simulink model "controllo_cartesiano"  (R2020b)
settings: Solver=VariableStepAuto  StartTime=0.0  StopTime=10.0  RelTol=1e-3
values from neighbouring files (symbols this model uses):
  f_G1 =     [workspaceMassaGravitaCoriolis.mat]
  f_G2 =     [workspaceMassaGravitaCoriolis.mat]
  f_G3 =     [workspaceMassaGravitaCoriolis.mat]
  f_M11 =     [workspaceMassaGravitaCoriolis.mat]
  f_M12 =     [workspaceMassaGravitaCoriolis.mat]
  f_M13 =     [workspaceMassaGravitaCoriolis.mat]
  f_M21 =     [workspaceMassaGravitaCoriolis.mat]
  f_M22 =     [workspaceMassaGravitaCoriolis.mat]
  f_M23 =     [workspaceMassaGravitaCoriolis.mat]
  f_M31 =     [workspaceMassaGravitaCoriolis.mat]
  f_M32 =     [workspaceMassaGravitaCoriolis.mat]
  f_M33 =     [workspaceMassaGravitaCoriolis.mat]
  f_V1 =     [workspaceMassaGravitaCoriolis.mat]
  f_V2 =     [workspaceMassaGravitaCoriolis.mat]
  f_V3 =     [workspaceMassaGravitaCoriolis.mat]
libraries: robotcorelib x1
(part 5 of 5)

== matlab function controllo_cartesiano/J ==
  data: Q input; dx output; dQ input; parametri input
function dx = J(Q,dQ,parametri)
l=parametri(1);
% d=parametri(2);
% m1=parametri(3);
% ma=parametri(4);
xc1=Q(1);
xc5=Q(2);
q2=Q(3);

J =[...
 
(l*sin(2*atan((2*l^2*sin(q2) + (3*l^4 + 4*cos(q2)*l^3*xc1 - 4*sin(q2)*l^3*xc5 - 2*cos(2*q2)*l^2*xc1^2 + 4*sin(2*q2)*l^2*xc1*xc5 + 2*cos(2*q2)*l^2*xc5^2 - 4*cos(q2)*l*xc1^3 + 4*sin(q2)*l*xc1^2*xc5 - 4*cos(q2)*l*xc1*xc5^2 + 4*sin(q2)*l*xc5^3 - xc1^4 - 2*xc1^2*xc5^2 - xc5^4)^(1/2) - 2*l*xc5)/(l^2 - 2*l*xc1 + xc1^2 + xc5^2 - 2*l^2*cos(q2) + 2*l*xc1*cos(q2) - 2*l*xc5*sin(q2))))*(((2*xc1 - 2*l + 2*l*cos(q2))*(2*l^2*sin(q2) + (3*l^4 + 4*cos(q2)*l^3*xc1 - 4*sin(q2)*l^3*xc5 - 2*cos(2*q2)*l^2*xc1^2 + 4*sin(2*q2)*l^2*xc1*xc5 + 2*cos(2*q2)*l^2*xc5^2 - 4*cos(q2)*l*xc1^3 + 4*sin(q2)*l*xc1^2*xc5 - 4*cos(q2)*l*xc1*xc5^2 + 4*sin(q2)*l*xc5^3 - xc1^4 - 2*xc1^2*xc5^2 - xc5^4)^(1/2) - 2*l*xc5))/(l^2 - 2*l*xc1 + xc1^2 + xc5^2 - 2*l^2*cos(q2) + 2*l*xc1*cos(q2) - 2*l*xc5*sin(q2))^2 + (2*(xc1 + l*cos(q2))*(- l^2 + 2*cos(q2)*l*xc1 - 2*sin(q2)*l*xc5 + xc1^2 + xc5^2))/((l^2 - 2*l*xc1 + xc1^2 + xc5^2 - 2*l^2*cos(q2) + 2*l*xc1*cos(q2) - 2*l*xc5*sin(q2))*(3*l^4 + 4*cos(q2)*l^3*xc1 - 4*sin(q2)*l^3*xc5 - 2*cos(2*q2)*l^2*xc1^2 + 4*sin(2*q2)*l^2*xc1*xc5 + 2*cos(2*q2)*l^2*xc5^2 - 4*cos(q2)*l*xc1^3 + 4*sin(q2)*l*xc1^2*xc5 - 4*cos(q2)*l*xc1*xc5^2 + 4*sin(q2)*l*xc5^3 - xc1^4 - 2*xc1^2*xc5^2 - xc5^4)^(1/2))))/((2*l^2*sin(q2) + (3*l^4 + 4*cos(q2)*l^3*xc1 - 4*sin(q2)*l^3*xc5 - 2*cos(2*q2)*l^2*xc1^2 + 4*sin(2*q2)*l^2*xc1*xc5 + 2*cos(2*q2)*l^2*xc5^2 - 4*cos(q2)*l*xc1^3 + 4*sin(q2)*l*xc1^2*xc5 - 4*cos(q2)*l*xc1*xc5^2 + 4*sin(q2)*l*xc5^3 - xc1^4 - 2*xc1^2*xc5^2 - xc5^4)^(1/2) - 2*l*xc5)^2/(l^2 - 2*l*xc1 + xc1^2 + xc5^2 - 2*l^2*cos(q2) + 2*l*xc1*cos(q2) - 2*l*xc5*sin(q2))^2 + 1) + 1, (l*sin(2*atan((2*l^2*sin(q2) + (3*l^4 + 4*cos(q2)*l^3*xc1 - 4*sin(q2)*l^3*xc5 - 2*cos(2*q2)*l^2*xc1^2 + 4*sin(2*q2)*l^2*xc1*xc5 + 2*cos(2*q2)*l^2*xc5^2 - 4*cos(q2)*l*xc1^3 + 4*sin(q2)*l*xc1^2*xc5 - 4*cos(q2)*l*xc1*xc5^2 + 4*sin(q2)*l*xc5^3 - xc1^4 - 2*xc1^2*xc5^2 - xc5^4)^(1/2) - 2*l*xc5)/(l^2 - 2*l*xc1 + xc1^2 + xc5^2 - 2*l^2*cos(q2) + 2*l*xc1*cos(q2) - 2*l*xc5*sin(q2))))*((2*l + (2*sin(q2)*l^3 - 2*sin(2*q2)*l^2*xc1 - 2*cos(2*q2)*l^2*xc5 - 2*sin(q2)*l*xc1^2 + 4*cos(q2)*l*xc1*xc5 - 6*sin(q2)*l*xc5^2 + 2*xc1^2*xc5 + 2*xc5^3)/(3*l^4 + 4*cos(q2)*l^3*xc1 - 4*sin(q2)*l^3*xc5 - 2*cos(2*q2)*l^2*xc1^2 + 4*sin(2*q2)*l^2*xc1*xc5 + 2*cos(2*q2)*l^2*xc5^2 - 4*cos(q2)*l*xc1^3 + 4*sin(q2)*l*xc1^2*xc5 - 4*cos(q2)*l*xc1*xc5^2 + 4*sin(q2)*l*xc5^3 - xc1^4 - 2*xc1^2*xc5^2 - xc5^4)^(1/2))/(l^2 - 2*l*xc1 + xc1^2 + xc5^2 - 2*l^2*cos(q2) + 2*l*xc1*cos(q2) - 2*l*xc5*sin(q2)) + ((2*xc5 - 2*l*sin(q2))*(2*l^2*sin(q2) + (3*l^4 + 4*cos(q2)*l^3*xc1 - 4*sin(q2)*l^3*xc5 - 2*cos(2*q2)*l^2*xc1^2 + 4*sin(2*q2)*l^2*xc1*xc5 + 2*cos(2*q2)*l^2*xc5^2 - 4*cos(q2)*l*xc1^3 + 4*sin(q2)*l*xc1^2*xc5 - 4*cos(q2)*l*xc1*xc5^2 + 4*sin(q2)*l*xc5^3 - xc1^4 - 2*xc1^2*xc5^2 - xc5^4)^(1/2) - 2*l*xc5))/(l^2 - 2*l*xc1 + xc1^2 + xc5^2 - 2*l^2*cos(q2) + 2*l*xc1*cos(q2) - 2*l*xc5*sin(q2))^2))/((2*l^2*sin(q2) + (3*l^4 + 4*cos(q2)*l^3*xc1 - 4*sin(q2)*l^3*xc5 - 2*cos(2*q2)*l^2*xc1^2 + 4*sin(2*q2)*l^2*xc1*xc5 + 2*cos(2*q2)*l^2*xc5^2 - 4*cos(q2)*l*xc1^3 + 4*sin(q2)*l*xc1^2*xc5 - 4*cos(q2)*l*xc1*xc5^2 + 4*sin(q2)*l*xc5^3 - xc1^4 - 2*xc1^2*xc5^2 - xc5^4)^(1/2) - 2*l*xc5)^2/(l^2 - 2*l*xc1 + xc1^2 + xc5^2 - 2*l^2*cos(q2) + 2*l*xc1*cos(q2) - 2*l*xc5*sin(q2))^2 + 1), - l*sin(q2) - (l*sin(2*atan((2*l^2*sin(q2) + (3*l^4 + 4*cos(q2)*l^3*xc1 - 4*sin(q2)*l^3*xc5 - 2*cos(2*q2)*l^2*xc1^2 + 4*sin(2*q2)*l^2*xc1*xc5 + 2*cos(2*q2)*l^2*xc5^2 - 4*cos(q2)*l*xc1^3 + 4*sin(q2)*l*xc1^2*xc5 - 4*cos(q2)*l*xc1*xc5^2 + 4*sin(q2)*l*xc5^3 - xc1^4 - 2*xc1^2*xc5^2 - xc5^4)^(1/2) - 2*l*xc5)/(l^2 - 2*l*xc1 + xc1^2 + xc5^2 - 2*l^2*cos(q2) + 2*l*xc1*cos(q2) - 2*l*xc5*sin(q2))))*((2*l^2*cos(q2) + (2*l*(- sin(q2)*l^2*xc1 - cos(q2)*l^2*xc5 + sin(2*q2)*l*xc1^2 + 2*cos(2*q2)*l*xc1*xc5 - sin(2*q2)*l*xc5^2 + sin(q2)*xc1^3 + cos(q2)*xc1^2*xc5 + sin(q2)*xc1*xc5^2 + cos(q2)*xc5^3))/(3*l^4 + 4*cos(q2)*l^3*xc1 - 4*sin(q2)*l^3*xc5 - 2*cos(2*q2)*l^2*xc1^2 + 4*sin(2*q2)*l^2*xc1*xc5 + 2*cos(2*q2)*l^2*xc5^2 - 4*cos(q2)*l*xc1^3 + 4*sin(q2)*l*xc1^2*xc5 - 4*cos(q2)*l*xc1*xc5^2 + 4*sin(q2)*l*xc5^3 - xc1^4 - 2*xc1^2*xc5^2 - xc5^4)^(1/2))/(l^2 - 2*l*xc1 + xc1^2 + xc5^2 - 2*l^2*cos(q2) + 2*l*xc1*cos(q2) - 2*l*xc5*sin(q2)) + (2*l*(xc5*cos(q2) - l*sin(q2) + xc1*sin(q2))*(2*l^2*sin(q2) + (3*l^4 + 4*cos(q2)*l^3*xc1 - 4*sin(q2)*l^3*xc5 - 2*cos(2*q2)*l^2*xc1^2 + 4*sin(2*q2)*l^2*xc1*xc5 + 2*cos(2*q2)*l^2*xc5^2 - 4*cos(q2)*l*xc1^3 + 4*sin(q2)*l*xc1^2*xc5 - 4*cos(q2)*l*xc1*xc5^2 + 4*sin(q2)*l*xc5^3 - xc1^4 - 2*xc1^2*xc5^2 - xc5^4)^(1/2) - 2*l*xc5))/(l^2 - 2*l*xc1 + xc1^2 + xc5^2 - 2*l^2*cos(q2) + 2*l*xc1*cos(q2) - 2*l*xc5*sin(q2))^2))/((2*l^2*sin(q2) + (3*l^4 + 4*cos(q2)*l^3*xc1 - 4*sin(q2)*l^3*xc5 - 2*cos(2*q2)*l^2*xc1^2 + 4*sin(2*q2)*l^2*xc1*xc5 + 2*cos(2*q2)*l^2*xc5^2 - 4*cos(q2)*l*xc1^3 + 4*sin(q2)*l*xc1^2*xc5 - 4*cos(q2)*l*xc1*xc5^2 + 4*sin(q2)*l*xc5^3 - xc1^4 - 2*xc1^2*xc5^2 - xc5^4)^(1/2) - 2*l*xc5)^2/(l^2 - 2*l*xc1 + xc1^2 + xc5^2 - 2*l^2*cos(q2) + 2*l*xc1*cos(q2) - 2*l*xc5*sin(q2))^2 + 1);...
    (l*cos(2*atan((2*l^2*sin(q2) + (3*l^4 + 4*cos(q2)*l^3*xc1 - 4*sin(q2)*l^3*xc5 - 2*cos(2*q2)*l^2*xc1^2 + 4*sin(2*q2)*l^2*xc1*xc5 + 2*cos(2*q2)*l^2*xc5^2 - 4*cos(q2)*l*xc1^3 + 4*sin(q2)*l*xc1^2*xc5 - 4*cos(q2)*l*xc1*xc5^2 + 4*sin(q2)*l*xc5^3 - xc1^4 - 2*xc1^2*xc5^2 - xc5^4)^(1/2) - 2*l*xc5)/(l^2 - 2*l*xc1 + xc1^2 + xc5^2 - 2*l^2*cos(q2) + 2*l*xc1*cos(q2) - 2*l*xc5*sin(q2))))*(((2*xc1 - 2*l + 2*l*cos(q2))*(2*l^2*sin(q2) + (3*l^4 + 4*cos(q2)*l^3*xc1 - 4*sin(q2)*l^3*xc5 - 2*cos(2*q2)*l^2*xc1^2 + 4*sin(2*q2)*l^2*xc1*xc5 + 2*cos(2*q2)*l^2*xc5^2 - 4*cos(q2)*l*xc1^3 + 4*sin(q2)*l*xc1^2*xc5 - 4*cos(q2)*l*xc1*xc5^2 + 4*sin(q2)*l*xc5^3 - xc1^4 - 2*xc1^2*xc5^2 - xc5^4)^(1/2) - 2*l*xc5))/(l^2 - 2*l*xc1 + xc1^2 + xc5^2 - 2*l^2*cos(q2) + 2*l*xc1*cos(q2) - 2*l*xc5*sin(q2))^2 + (2*(xc1 + l*cos(q2))*(- l^2 + 2*cos(q2)*l*xc1 - 2*sin(q2)*l*xc5 + xc1^2 + xc5^2))/((l^2 - 2*l*xc1 + xc1^2 + xc5^2 - 2*l^2*cos(q2) + 2*l*xc1*cos(q2) - 2*l*xc5*sin(q2))*(3*l^4 + 4*cos(q2)*l^3*xc1 - 4*sin(q2)*l^3*xc5 - 2*cos(2*q2)*l^2*xc1^2 + 4*sin(2*q2)*l^2*xc1*xc5 + 2*cos(2*q2)*l^2*xc5^2 - 4*cos(q2)*l*xc1^3 + 4*sin(q2)*l*xc1^2*xc5 - 4*cos(q2)*l*xc1*xc5^2 + 4*sin(q2)*l*xc5^3 - xc1^4 - 2*xc1^2*xc5^2 - xc5^4)^(1/2))))/((2*l^2*sin(q2) + (3*l^4 + 4*cos(q2)*l^3*xc1 - 4*sin(q2)*l^3*xc5 - 2*cos(2*q2)*l^2*xc1^2 + 4*sin(2*q2)*l^2*xc1*xc5 + 2*cos(2*q2)*l^2*xc5^2 - 4*cos(q2)*l*xc1^3 + 4*sin(q2)*l*xc1^2*xc5 - 4*cos(q2)*l*xc1*xc5^2 + 4*sin(q2)*l*xc5^3 - xc1^4 - 2*xc1^2*xc5^2 - xc5^4)^(1/2) - 2*l*xc5)^2/(l^2 - 2*l*xc1 + xc1^2 + xc5^2 - 2*l^2*cos(q2) + 2*l*xc1*cos(q2) - 2*l*xc5*sin(q2))^2 + 1), (l*cos(2*atan((2*l^2*sin(q2) + (3*l^4 + 4*cos(q2)*l^3*xc1 - 4*sin(q2)*l^3*xc5 - 2*cos(2*q2)*l^2*xc1^2 + 4*sin(2*q2)*l^2*xc1*xc5 + 2*cos(2*q2)*l^2*xc5^2 - 4*cos(q2)*l*xc1^3 + 4*sin(q2)*l*xc1^2*xc5 - 4*cos(q2)*l*xc1*xc5^2 + 4*sin(q2)*l*xc5^3 - xc1^4 - 2*xc1^2*xc5^2 - xc5^4)^(1/2) - 2*l*xc5)/(l^2 - 2*l*xc1 + xc1^2 + xc5^2 - 2*l^2*cos(q2) + 2*l*xc1*cos(q2) - 2*l*xc5*sin(q2))))*((2*l + (2*sin(q2)*l^3 - 2*sin(2*q2)*l^2*xc1 - 2*cos(2*q2)*l^2*xc5 - 2*sin(q2)*l*xc1^2 + 4*cos(q2)*l*xc1*xc5 - 6*sin(q2)*l*xc5^2 + 2*xc1^2*xc5 + 2*xc5^3)/(3*l^4 + 4*cos(q2)*l^3*xc1 - 4*sin(q2)*l^3*xc5 - 2*cos(2*q2)*l^2*xc1^2 + 4*sin(2*q2)*l^2*xc1*xc5 + 2*cos(2*q2)*l^2*xc5^2 - 4*cos(q2)*l*xc1^3 + 4*sin(q2)*l*xc1^2*xc5 - 4*cos(q2)*l*xc1*xc5^2 + 4*sin(q2)*l*xc5^3 - xc1^4 - 2*xc1^2*xc5^2 - xc5^4)^(1/2))/(l^2 - 2*l*xc1 + xc1^2 + xc5^2 - 2*l^2*cos(q2) + 2*l*xc1*cos(q2) - 2*l*xc5*sin(q2)) + ((2*xc5 - 2*l*sin(q2))*(2*l^2*sin(q2) + (3*l^4 + 4*cos(q2)*l^3*xc1 - 4*sin(q2)*l^3*xc5 - 2*cos(2*q2)*l^2*xc1^2 + 4*sin(2*q2)*l^2*xc1*xc5 + 2*cos(2*q2)*l^2*xc5^2 - 4*cos(q2)*l*xc1^3 + 4*sin(q2)*l*xc1^2*xc5 - 4*cos(q2)*l*xc1*xc5^2 + 4*sin(q2)*l*xc5^3 - xc1^4 - 2*xc1^2*xc5^2 - xc5^4)^(1/2) - 2*l*xc5))/(l^2 - 2*l*xc1 + xc1^2 + xc5^2 - 2*l^2*cos(q2) + 2*l*xc1*cos(q2) - 2*l*xc5*sin(q2))^2))/((2*l^2*sin(q2) + (3*l^4 + 4*cos(q2)*l^3*xc1 - 4*sin(q2)*l^3*xc5 - 2*cos(2*q2)*l^2*xc1^2 + 4*sin(2*q2)*l^2*xc1*xc5 + 2*cos(2*q2)*l^2*xc5^2 - 4*cos(q2)*l*xc1^3 + 4*sin(q2)*l*xc1^2*xc5 - 4*cos(q2)*l*xc1*xc5^2 + 4*sin(q2)*l*xc5^3 - xc1^4 - 2*xc1^2*xc5^2 - xc5^4)^(1/2) - 2*l*xc5)^2/(l^2 - 2*l*xc1 + xc1^2 + xc5^2 - 2*l^2*cos(q2) + 2*l*xc1*cos(q2) - 2*l*xc5*sin(q2))^2 + 1),   l*cos(q2) - (l*cos(2*atan((2*l^2*sin(q2) + (3*l^4 + 4*cos(q2)*l^3*xc1 - 4*sin(q2)*l^3*xc5 - 2*cos(2*q2)*l^2*xc1^2 + 4*sin(2*q2)*l^2*xc1*xc5 + 2*cos(2*q2)*l^2*xc5^2 - 4*cos(q2)*l*xc1^3 + 4*sin(q2)*l*xc1^2*xc5 - 4*cos(q2)*l*xc1*xc5^2 + 4*sin(q2)*l*xc5^3 - xc1^4 - 2*xc1^2*xc5^2 - xc5^4)^(1/2) - 2*l*xc5)/(l^2 - 2*l*xc1 + xc1^2 + xc5^2 - 2*l^2*cos(q2) + 2*l*xc1*cos(q2) - 2*l*xc5*sin(q2))))*((2*l^2*cos(q2) + (2*l*(- sin(q2)*l^2*xc1 - cos(q2)*l^2*xc5 + sin(2*q2)*l*xc1^2 + 2*cos(2*q2)*l*xc1*xc5 - sin(2*q2)*l*xc5^2 + sin(q2)*xc1^3 + cos(q2)*xc1^2*xc5 + sin(q2)*xc1*xc5^2 + cos(q2)*xc5^3))/(3*l^4 + 4*cos(q2)*l^3*xc1 - 4*sin(q2)*l^3*xc5 - 2*cos(2*q2)*l^2*xc1^2 + 4*sin(2*q2)*l^2*xc1*xc5 + 2*cos(2*q2)*l^2*xc5^2 - 4*cos(q2)*l*xc1^3 + 4*sin(q2)*l*xc1^2*xc5 - 4*cos(q2)*l*xc1*xc5^2 + 4*sin(q2)*l*xc5^3 - xc1^4 - 2*xc1^2*xc5^2 - xc5^4)^(1/2))/(l^2 - 2*l*xc1 + xc1^2 + xc5^2 - 2*l^2*cos(q2) + 2*l*xc1*cos(q2) - 2*l*xc5*sin(q2)) + (2*l*(xc5*cos(q2) - l*sin(q2) + xc1*sin(q2))*(2*l^2*sin(q2) + (3*l^4 + 4*cos(q2)*l^3*xc1 - 4*sin(q2)*l^3*xc5 - 2*cos(2*q2)*l^2*xc1^2 + 4*sin(2*q2)*l^2*xc1*xc5 + 2*cos(2*q2)*l^2*xc5^2 - 4*cos(q2)*l*xc1^3 + 4*sin(q2)*l*xc1^2*xc5 - 4*cos(q2)*l*xc1*xc5^2 + 4*sin(q2)*l*xc5^3 - xc1^4 - 2*xc1^2*xc5^2 - xc5^4)^(1/2) - 2*l*xc5))/(l^2 - 2*l*xc1 + xc1^2 + xc5^2 - 2*l^2*cos(q2) + 2*l*xc1*cos(q2) - 2*l*xc5*sin(q2))^2))/((2*l^2*sin(q2) + (3*l^4 + 4*cos(q2)*l^3*xc1 - 4*sin(q2)*l^3*xc5 - 2*cos(2*q2)*l^2*xc1^2 + 4*sin(2*q2)*l^2*xc1*xc5 + 2*cos(2*q2)*l^2*xc5^2 - 4*cos(q2)*l*xc1^3 + 4*sin(q2)*l*xc1^2*xc5 - 4*cos(q2)*l*xc1*xc5^2 + 4*sin(q2)*l*xc5^3 - xc1^4 - 2*xc1^2*xc5^2 - xc5^4)^(1/2) - 2*l*xc5)^2/(l^2 - 2*l*xc1 + xc1^2 + xc5^2 - 2*l^2*cos(q2) + 2*l*xc1*cos(q2) - 2*l*xc5*sin(q2))^2 + 1);...
                                                                                                                                                                                                                                                                                                                                                                                         (2*(((2*xc1 - 2*l + 2*l*cos(q2))*(2*l^2*sin(q2) + (3*l^4 + 4*cos(q2)*l^3*xc1 - 4*sin(q2)*l^3*xc5 - 2*cos(2*q2)*l^2*xc1^2 + 4*sin(2*q2)*l^2*xc1*xc5 + 2*cos(2*q2)*l^2*xc5^2 - 4*cos(q2)*l*xc1^3 + 4*sin(q2)*l*xc1^2*xc5 - 4*cos(q2)*l*xc1*xc5^2 + 4*sin(q2)*l*xc5^3 - xc1^4 - 2*xc1^2*xc5^2 - xc5^4)^(1/2) - 2*l*xc5))/(l^2 - 2*l*xc1 + xc1^2 + xc5^2 - 2*l^2*cos(q2) + 2*l*xc1*cos(q2) - 2*l*xc5*sin(q2))^2 + (2*(xc1 + l*cos(q2))*(- l^2 + 2*cos(q2)*l*xc1 - 2*sin(q2)*l*xc5 + xc1^2 + xc5^2))/((l^2 - 2*l*xc1 + xc1^2 + xc5^2 - 2*l^2*cos(q2) + 2*l*xc1*cos(q2) - 2*l*xc5*sin(q2))*(3*l^4 + 4*cos(q2)*l^3*xc1 - 4*sin(q2)*l^3*xc5 - 2*cos(2*q2)*l^2*xc1^2 + 4*sin(2*q2)*l^2*xc1*xc5 + 2*cos(2*q2)*l^2*xc5^2 - 4*cos(q2)*l*xc1^3 + 4*sin(q2)*l*xc1^2*xc5 - 4*cos(q2)*l*xc1*xc5^2 + 4*sin(q2)*l*xc5^3 - xc1^4 - 2*xc1^2*xc5^2 - xc5^4)^(1/2))))/((2*l^2*sin(q2) + (3*l^4 + 4*cos(q2)*l^3*xc1 - 4*sin(q2)*l^3*xc5 - 2*cos(2*q2)*l^2*xc1^2 + 4*sin(2*q2)*l^2*xc1*xc5 + 2*cos(2*q2)*l^2*xc5^2 - 4*cos(q2)*l*xc1^3 + 4*sin(q2)*l*xc1^2*xc5 - 4*cos(q2)*l*xc1*xc5^2 + 4*sin(q2)*l*xc5^3 - xc1^4 - 2*xc1^2*xc5^2 - xc5^4)^(1/2) - 2*l*xc5)^2/(l^2 - 2*l*xc1 + xc1^2 + xc5^2 - 2*l^2*cos(q2) + 2*l*xc1*cos(q2) - 2*l*xc5*sin(q2))^2 + 1),                                                                                                                                                                                                                                                                                                                                                                                      (2*((2*l + (2*sin(q2)*l^3 - 2*sin(2*q2)*l^2*xc1 - 2*cos(2*q2)*l^2*xc5 - 2*sin(q2)*l*xc1^2 + 4*cos(q2)*l*xc1*xc5 - 6*sin(q2)*l*xc5^2 + 2*xc1^2*xc5 + 2*xc5^3)/(3*l^4 + 4*cos(q2)*l^3*xc1 - 4*sin(q2)*l^3*xc5 - 2*cos(2*q2)*l^2*xc1^2 + 4*sin(2*q2)*l^2*xc1*xc5 + 2*cos(2*q2)*l^2*xc5^2 - 4*cos(q2)*l*xc1^3 + 4*sin(q2)*l*xc1^2*xc5 - 4*cos(q2)*l*xc1*xc5^2 + 4*sin(q2)*l*xc5^3 - xc1^4 - 2*xc1^2*xc5^2 - xc5^4)^(1/2))/(l^2 - 2*l*xc1 + xc1^2 + xc5^2 - 2*l^2*cos(q2) + 2*l*xc1*cos(q2) - 2*l*xc5*sin(q2)) + ((2*xc5 - 2*l*sin(q2))*(2*l^2*sin(q2) + (3*l^4 + 4*cos(q2)*l^3*xc1 - 4*sin(q2)*l^3*xc5 - 2*cos(2*q2)*l^2*xc1^2 + 4*sin(2*q2)*l^2*xc1*xc5 + 2*cos(2*q2)*l^2*xc5^2 - 4*cos(q2)*l*xc1^3 + 4*sin(q2)*l*xc1^2*xc5 - 4*cos(q2)*l*xc1*xc5^2 + 4*sin(q2)*l*xc5^3 - xc1^4 - 2*xc1^2*xc5^2 - xc5^4)^(1/2) - 2*l*xc5))/(l^2 - 2*l*xc1 + xc1^2 + xc5^2 - 2*l^2*cos(q2) + 2*l*xc1*cos(q2) - 2*l*xc5*sin(q2))^2))/((2*l^2*sin(q2) + (3*l^4 + 4*cos(q2)*l^3*xc1 - 4*sin(q2)*l^3*xc5 - 2*cos(2*q2)*l^2*xc1^2 + 4*sin(2*q2)*l^2*xc1*xc5 + 2*cos(2*q2)*l^2*xc5^2 - 4*cos(q2)*l*xc1^3 + 4*sin(q2)*l*xc1^2*xc5 - 4*cos(q2)*l*xc1*xc5^2 + 4*sin(q2)*l*xc5^3 - xc1^4 - 2*xc1^2*xc5^2 - xc5^4)^(1/2) - 2*l*xc5)^2/(l^2 - 2*l*xc1 + xc1^2 + xc5^2 - 2*l^2*cos(q2) + 2*l*xc1*cos(q2) - 2*l*xc5*sin(q2))^2 + 1),                                                                                                                                                                                                                                                                                                                                                                                                   -(2*((2*l^2*cos(q2) + (2*l*(- sin(q2)*l^2*xc1 - cos(q2)*l^2*xc5 + sin(2*q2)*l*xc1^2 + 2*cos(2*q2)*l*xc1*xc5 - sin(2*q2)*l*xc5^2 + sin(q2)*xc1^3 + cos(q2)*xc1^2*xc5 + sin(q2)*xc1*xc5^2 + cos(q2)*xc5^3))/(3*l^4 + 4*cos(q2)*l^3*xc1 - 4*sin(q2)*l^3*xc5 - 2*cos(2*q2)*l^2*xc1^2 + 4*sin(2*q2)*l^2*xc1*xc5 + 2*cos(2*q2)*l^2*xc5^2 - 4*cos(q2)*l*xc1^3 + 4*sin(q2)*l*xc1^2*xc5 - 4*cos(q2)*l*xc1*xc5^2 + 4*sin(q2)*l*xc5^3 - xc1^4 - 2*xc1^2*xc5^2 - xc5^4)^(1/2))/(l^2 - 2*l*xc1 + xc1^2 + xc5^2 - 2*l^2*cos(q2) + 2*l*xc1*cos(q2) - 2*l*xc5*sin(q2)) + (2*l*(xc5*cos(q2) - l*sin(q2) + xc1*sin(q2))*(2*l^2*sin(q2) + (3*l^4 + 4*cos(q2)*l^3*xc1 - 4*sin(q2)*l^3*xc5 - 2*cos(2*q2)*l^2*xc1^2 + 4*sin(2*q2)*l^2*xc1*xc5 + 2*cos(2*q2)*l^2*xc5^2 - 4*cos(q2)*l*xc1^3 + 4*sin(q2)*l*xc1^2*xc5 - 4*cos(q2)*l*xc1*xc5^2 + 4*sin(q2)*l*xc5^3 - xc1^4 - 2*xc1^2*xc5^2 - xc5^4)^(1/2) - 2*l*xc5))/(l^2 - 2*l*xc1 + xc1^2 + xc5^2 - 2*l^2*cos(q2) + 2*l*xc1*cos(q2) - 2*l*xc5*sin(q2))^2))/((2*l^2*sin(q2) + (3*l^4 + 4*cos(q2)*l^3*xc1 - 4*sin(q2)*l^3*xc5 - 2*cos(2*q2)*l^2*xc1^2 + 4*sin(2*q2)*l^2*xc1*xc5 + 2*cos(2*q2)*l^2*xc5^2 - 4*cos(q2)*l*xc1^3 + 4*sin(q2)*l*xc1^2*xc5 - 4*cos(q2)*l*xc1*xc5^2 + 4*sin(q2)*l*xc5^3 - xc1^4 - 2*xc1^2*xc5^2 - xc5^4)^(1/2) - 2*l*xc5)^2/(l^2 - 2*l*xc1 + xc1^2 + xc5^2 - 2*l^2*cos(q2) + 2*l*xc1*cos(q2) - 2*l*xc5*sin(q2))^2 + 1)];

dx=J*dQ;
end

== matlab function controllo_cartesiano/kin_dir1 ==
  data: Q input; P output; parametri input
function P  = kin_dir_pos(Q,parametri) %P[X Y alpha]
l=parametri(1);
d=parametri(2);
m1=parametri(3);
ma=parametri(4);
xc1=Q(1);
xc5=Q(2);
q2=Q(3);


q3 = ...
 -q2 - 2*atan((2*l*xc5 + (-(2*l*xc1 + l^2 + l^2*tan(q2/2)^2 + xc1^2 + xc5^2 + xc1^2*tan(q2/2)^2 + xc5^2*tan(q2/2)^2 - 4*l*xc5*tan(q2/2) - 2*l*xc1*tan(q2/2)^2)*(2*l*xc1 - 3*l^2 - 3*l^2*tan(q2/2)^2 + xc1^2 + xc5^2 + xc1^2*tan(q2/2)^2 + xc5^2*tan(q2/2)^2 - 4*l*xc5*tan(q2/2) - 2*l*xc1*tan(q2/2)^2))^(1/2) - 4*l^2*tan(q2/2) + 2*l*xc5*tan(q2/2)^2)/(3*l^2*tan(q2/2)^2 - l^2 + xc1^2 + xc5^2 + xc1^2*tan(q2/2)^2 + xc5^2*tan(q2/2)^2 - 4*l*xc5*tan(q2/2) - 4*l*xc1*tan(q2/2)^2) - (4*(l*xc5 - 2*l^2*tan(q2/2) + l*xc5*tan(q2/2)^2))/(3*l^2*tan(q2/2)^2 - l^2 + xc1^2 + xc5^2 + xc1^2*tan(q2/2)^2 + xc5^2*tan(q2/2)^2 - 4*l*xc5*tan(q2/2) - 4*l*xc1*tan(q2/2)^2));
q4 = ...
2*atan((2*l*xc5 + (-(2*l*xc1 + l^2 + l^2*tan(q2/2)^2 + xc1^2 + xc5^2 + xc1^2*tan(q2/2)^2 + xc5^2*tan(q2/2)^2 - 4*l*xc5*tan(q2/2) - 2*l*xc1*tan(q2/2)^2)*(2*l*xc1 - 3*l^2 - 3*l^2*tan(q2/2)^2 + xc1^2 + xc5^2 + xc1^2*tan(q2/2)^2 + xc5^2*tan(q2/2)^2 - 4*l*xc5*tan(q2/2) - 2*l*xc1*tan(q2/2)^2))^(1/2) - 4*l^2*tan(q2/2) + 2*l*xc5*tan(q2/2)^2)/(3*l^2*tan(q2/2)^2 - l^2 + xc1^2 + xc5^2 + xc1^2*tan(q2/2)^2 + xc5^2*tan(q2/2)^2 - 4*l*xc5*tan(q2/2) - 4*l*xc1*tan(q2/2)^2)) + 2*atan((2*l*xc5 + (-(2*l*xc1 + l^2 + l^2*tan(q2/2)^2 + xc1^2 + xc5^2 + xc1^2*tan(q2/2)^2 + xc5^2*tan(q2/2)^2 - 4*l*xc5*tan(q2/2) - 2*l*xc1*tan(q2/2)^2)*(2*l*xc1 - 3*l^2 - 3*l^2*tan(q2/2)^2 + xc1^2 + xc5^2 + xc1^2*tan(q2/2)^2 + xc5^2*tan(q2/2)^2 - 4*l*xc5*tan(q2/2) - 2*l*xc1*tan(q2/2)^2))^(1/2) - 4*l^2*tan(q2/2) + 2*l*xc5*tan(q2/2)^2)/(3*l^2*tan(q2/2)^2 - l^2 + xc1^2 + xc5^2 + xc1^2*tan(q2/2)^2 + xc5^2*tan(q2/2)^2 - 4*l*xc5*tan(q2/2) - 4*l*xc1*tan(q2/2)^2) - (4*(l*xc5 - 2*l^2*tan(q2/2) + l*xc5*tan(q2/2)^2))/(3*l^2*tan(q2/2)^2 - l^2 + xc1^2 + xc5^2 + xc1^2*tan(q2/2)^2 + xc5^2*tan(q2/2)^2 - 4*l*xc5*tan(q2/2) - 4*l*xc1*tan(q2/2)^2));


gamma = q2+q3;
%beta = q2+q3+q4;
alpha=gamma-pi/2;

P=zeros(3,1);
P(1) = xc1+l*cos(q2)+l/2*cos(gamma)+d*cos(alpha);
P(2) = l*sin(q2)+l/2*sin(gamma)+d*sin(alpha);
P(3) = q2 + q3 - pi/2;

end

== matlab function controllo_cartesiano/Inerzie1 ==
  data: parametri input; I output
function I = Inerzie(parametri)
l=parametri(1);
d=parametri(2);
%m1=parametri(3);
ma=parametri(4);


I2 = ma*l^2/4 + 1/12 *ma*l^2;
I5 = I2;
I3 = I2 + 1/12 * ma*d^2 + ma*(d^2/4+l^2/4);
I=[I2;I5;I3];
end

== matlab function controllo_cartesiano/robot/massa_real/massa ==
  data: M output; Mij input
function  M= matrice_massa(Mij)

M=[Mij(1) Mij(2) Mij(3);Mij(4) Mij(5) Mij(6);Mij(7) Mij(8) Mij(9)];

end

== matlab function controllo_cartesiano/robot/robot ==
  data: M input; Q output; G input; V input; dt input; Q_prev input; dQ_prev input; dQ output; ddQ output; tau input
function [Q,dQ,ddQ] = robot(M,G,V,dt,Q_prev,dQ_prev,tau)
%ddq=inv(M)*(tau-N)  (N=V+G)
ddQ=M\(tau-V-G);
dQ=dQ_prev+ddQ*dt;
Q=Q_prev+dQ*dt;
end
